simulink model "Lab3_P2_atrito_variavel"  (R2020b)
settings: Solver=VariableStepAuto  StartTime=0.0  StopTime=8  MaxStep=0.5e-2  RelTol=1e-3
libraries: simulink x4
settings Model: Creator=rodsc  LastModifiedBy=rodsc
settings SolverCC: ZeroCrossAlgorithm=Adaptive
settings DebuggingCC: IgnoredZcDiagnostic=none

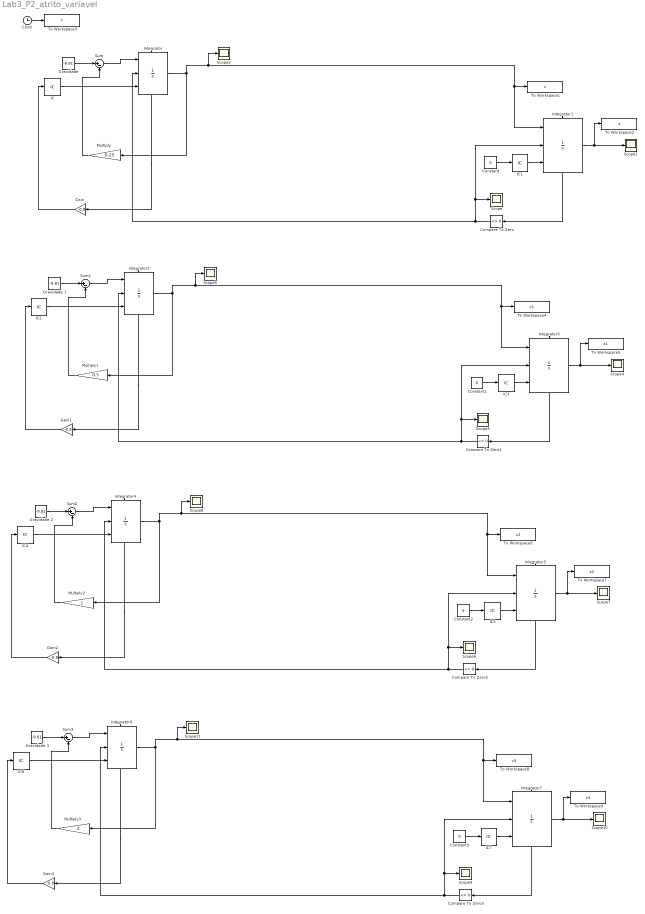
== system Lab3_P2_atrito_variavel ==
  Clock : Clock
  Compare To Zero{,1..3} (4 alike) : simulink/Logic and Bit Operations/Compare To Zero  relop=<=  OutDataTypeStr=boolean
  Constant{,1..3} (4 alike) : Constant  Value=0
  Gain{,1..3} (4 alike) : Gain  Gain=-0.8
  Gravidade {,1..3} (4 alike) : Constant  Value=-9.81
  IC{,2,4,6} (4 alike) : InitialCondition  Value=0
  IC1 : InitialCondition  Value=10
  IC3 : InitialCondition  Value=10
  IC5 : InitialCondition  Value=10
  IC7 : InitialCondition  Value=20
  Integrator{,2,4,6} (4 alike) : Integrator  ExternalReset=rising  InitialConditionSource=external  ShowStatePort=on
  Integrator{1,3,5,7} (4 alike) : Integrator  ExternalReset=rising  InitialConditionSource=external  LowerSaturationLimit=0  ShowStatePort=on
  Multiply : Gain  Gain=0.25
  Multiply1 : Gain  Gain=0.5
  Multiply2 : Gain
  Multiply3 : Gain  Gain=2
  Scope{,1..11} (12 alike) : Scope
  Sum{,1..3} (4 alike) : Sum  Inputs=|+-  OutMax=[0]
  To Workspace1 : ToWorkspace  VariableName=v  SampleTime=-1
      settings: Save2DSignal=2-D array (concatenate along first dimension)
  To Workspace2 : ToWorkspace  VariableName=z  SampleTime=-1
      settings: Save2DSignal=2-D array (concatenate along first dimension)
  To Workspace3 : ToWorkspace  VariableName=t  SampleTime=-1
      settings: Save2DSignal=2-D array (concatenate along first dimension)
  To Workspace4 : ToWorkspace  VariableName=v1  SampleTime=-1
      settings: Save2DSignal=2-D array (concatenate along first dimension)
  To Workspace5 : ToWorkspace  VariableName=z1  SampleTime=-1
      settings: Save2DSignal=2-D array (concatenate along first dimension)
  To Workspace6 : ToWorkspace  VariableName=v2  SampleTime=-1
      settings: Save2DSignal=2-D array (concatenate along first dimension)
  To Workspace7 : ToWorkspace  VariableName=z2  SampleTime=-1
      settings: Save2DSignal=2-D array (concatenate along first dimension)
  To Workspace8 : ToWorkspace  VariableName=v3  SampleTime=-1
      settings: Save2DSignal=2-D array (concatenate along first dimension)
  To Workspace9 : ToWorkspace  VariableName=z3  SampleTime=-1
      settings: Save2DSignal=2-D array (concatenate along first dimension)
  wires:
  IC/1 -> Integrator/3
  Integrator/1 -> Multiply/1, Scope2/1, Integrator1/1, To Workspace1/1
  Gain/1 -> IC/1
  Integrator/State -> Gain/1
  Integrator1/State -> Compare To Zero/1
  Compare To Zero/1 -> Integrator/2, Scope/1, Integrator1/2
  Constant/1 -> IC1/1
  IC1/1 -> Integrator1/3
  Integrator1/1 -> To Workspace2/1, Scope1/1
  Clock/1 -> To Workspace3/1
  "Gravidade "/1 -> Sum/1
  Sum/1 -> Integrator/1
  Multiply/1 -> Sum/2
  Gain1/1 -> IC2/1
  Integrator3/State -> Compare To Zero1/1
  Multiply1/1 -> Sum1/2
  Integrator2/State -> Gain1/1
  Sum1/1 -> Integrator2/1
  Integrator3/1 -> To Workspace5/1, Scope4/1
  Constant1/1 -> IC3/1
  IC3/1 -> Integrator3/3
  Gravidade 1/1 -> Sum1/1
  IC2/1 -> Integrator2/3
  Integrator2/1 -> Multiply1/1, Scope5/1, Integrator3/1, To Workspace4/1
  Compare To Zero1/1 -> Integrator2/2, Scope3/1, Integrator3/2
  Gain2/1 -> IC4/1
  Integrator5/State -> Compare To Zero2/1
  Multiply2/1 -> Sum2/2
  Integrator4/State -> Gain2/1
  Sum2/1 -> Integrator4/1
  Integrator5/1 -> To Workspace7/1, Scope7/1
  Constant2/1 -> IC5/1
  IC5/1 -> Integrator5/3
  Gravidade 2/1 -> Sum2/1
  IC4/1 -> Integrator4/3
  Integrator4/1 -> Multiply2/1, Scope8/1, Integrator5/1, To Workspace6/1
  Compare To Zero2/1 -> Integrator4/2, Scope6/1, Integrator5/2
  Gain3/1 -> IC6/1
  Integrator7/State -> Compare To Zero3/1
  Multiply3/1 -> Sum3/2
  Integrator6/State -> Gain3/1
  Sum3/1 -> Integrator6/1
  Integrator7/1 -> To Workspace9/1, Scope10/1
  Constant3/1 -> IC7/1
  IC7/1 -> Integrator7/3
  Gravidade 3/1 -> Sum3/1
  IC6/1 -> Integrator6/3
  Integrator6/1 -> Multiply3/1, Scope11/1, Integrator7/1, To Workspace8/1
  Compare To Zero3/1 -> Integrator6/2, Scope9/1, Integrator7/2
